simulink model "sim1"  (R2019b)
settings: Solver=VariableStepAuto  StartTime=0.0  StopTime=10.0  RelTol=1e-3
libraries: visionsources x2
settings Model: Creator=SAICHARAN  LastModifiedBy=vardhan
settings DataIOCC: ReturnWorkspaceOutputs=off
settings DebuggingCC: ArithmeticOperatorsInVariantConditions=warning
settings SFSimCC: SimUseLocalCustomCode=off  CustomCodeUndefinedFunction=UseInterfaceOnly
settings RTWCC: RTWUseLocalCustomCode=off

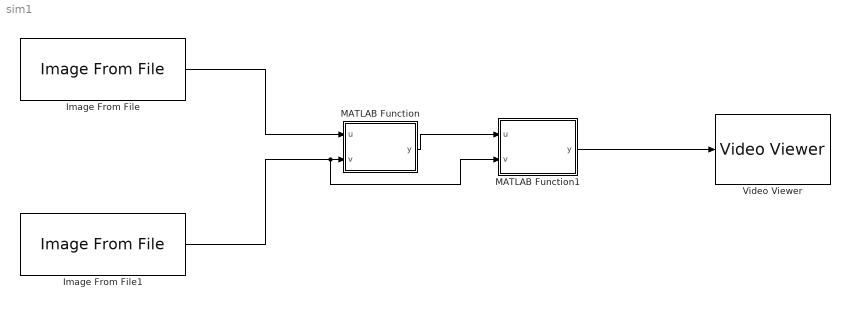
== system sim1 ==
  Image From File : visionsources/Image From File  Tag=vipblks_nd  FileName=C:\Users\SAICHARAN\Downloads\original.png  Ts=inf  imagePorts=One multidimensional signal  OutPortLabels=R|G|B  ImageDataType=Inherit from input image  sdImageDataType=uint(8)  Signed=on  WordLength=16  FractionLengthMode=User-defined  FractionLength=15
      settings: SourceProductName=Computer Vision Toolbox
  Image From File1 : visionsources/Image From File  Tag=vipblks_nd  FileName=C:\Users\SAICHARAN\Downloads\cameraman (1).tif  Ts=inf  imagePorts=One multidimensional signal  OutPortLabels=R|G|B  ImageDataType=Inherit from input image  sdImageDataType=uint(8)  Signed=on  WordLength=16  FractionLengthMode=User-defined  FractionLength=15
      settings: SourceProductName=Computer Vision Toolbox
  MATLAB Function : MATLAB Function  TreatAsAtomicUnit=on
  MATLAB Function1 : MATLAB Function  TreatAsAtomicUnit=on
  Video Viewer : VideoViewer  FigPos=[1116.33333333333 382 277.333333333333 129.333333333333]
  wires:
  MATLAB Function1/1(y) -> Video Viewer/1
  MATLAB Function/1(y) -> MATLAB Function1/1(u)
  Image From File/1 -> MATLAB Function/1(u)
  Image From File1/1 -> MATLAB Function1/2(v), MATLAB Function/2(v)

== matlab function sim1/MATLAB Function1 ==
  data: u input; y output; v input
function y = fcn(u,v)
coder.extrinsic('dct2');
coder.extrinsic('idct2');
dct_a = zeros(256,256);
dct_b = zeros(256,256);
c = zeros(256,256);
p = zeros(256,256);

dct_a = dct2(u);
dct_b = dct2(v);
c = dct_a - dct_b;

p = uint8(255 * c);
p = p(1:128,1:128);

y = p;

== matlab function sim1/MATLAB Function ==
  data: u input; y output; v input
function y = fcn(u,v)
coder.extrinsic('dct2');
coder.extrinsic('idct2');
dct_b = zeros(256,256);
idct_sum = zeros(256,256);
sum = zeros(256,256);

ba = imbinarize(u); % conversion of image into binary
[m,n]=size(ba);
a1 = [ba, zeros(256-m,256-n);zeros(256-m,256)]; % zero padding
dct_b = dct2(v);
sum = double(a1) + dct_b; % addition of two images
idct_sum = idct2(sum);
idct_sum = uint8(idct_sum);

%Error using imwrite (line 528)
%Unable to open file "hidden_img.png" for writing. You might not have
%write permission.
%Error in hideimg (line 19)
%imwrite(double(idct_sum),'hidden_img.png');

y = idct_sum;
